simulink model "ThreePhaseInductionMachine"  (R2022b)
settings: Solver=VariableStepAuto  StartTime=0.0  StopTime=5  MaxStep=25e-6  EnableMultiTasking=on
libraries: spsACVoltageSourceLib x3, spsControlledCurrentSourceLib x3, spsVoltageMeasurementLib x3, spsSeriesRLCBranchLib x3, spsdq0toabcLib x2, spsabctodq0Lib x1, spspowerguiLib x1
settings Model: Creator=James Green  LastModifiedBy=Sarthak M Desai
settings SolverCC: AlgebraicLoopSolver=TrustRegion
settings DataIOCC: ReturnWorkspaceOutputs=off
settings OptimizationCC: LifeSpan=inf
settings DebuggingCC: UnconnectedInputMsg=warning  UnconnectedOutputMsg=warning  UnconnectedLineMsg=warning  SFUnexpectedBacktrackingDiag=warning  SFNoUnconditionalDefaultTransitionDiag=warning  SFMachineParentedDataDiag=warning  ArithmeticOperatorsInVariantConditions=warning
settings ModelReferenceCC: EnableRefExpFcnMdlSchedulingChecks=on
settings SFSimCC: SimUseLocalCustomCode=off  CustomCodeUndefinedFunction=UseInterfaceOnly
settings RTWCC: RTWUseLocalCustomCode=off
settings CodeAppCC: StateflowObjectComments=on
settings GRTTargetCC: TargetLangStandard=C89/C90 (ANSI)
settings ConfigComp: CovMetricSettings=dw  CovSaveCumulativeToWorkspaceVar=on  CovSaveSingleToWorkspaceVar=on  CovExternalEMLEnable=off
settings SimscapeCC: SimscapeNormalizeSystem=off

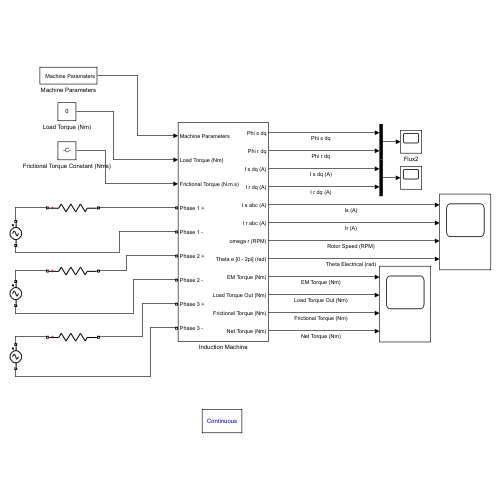
[thumbnail: Simulink's stored preview of the top-level diagram]
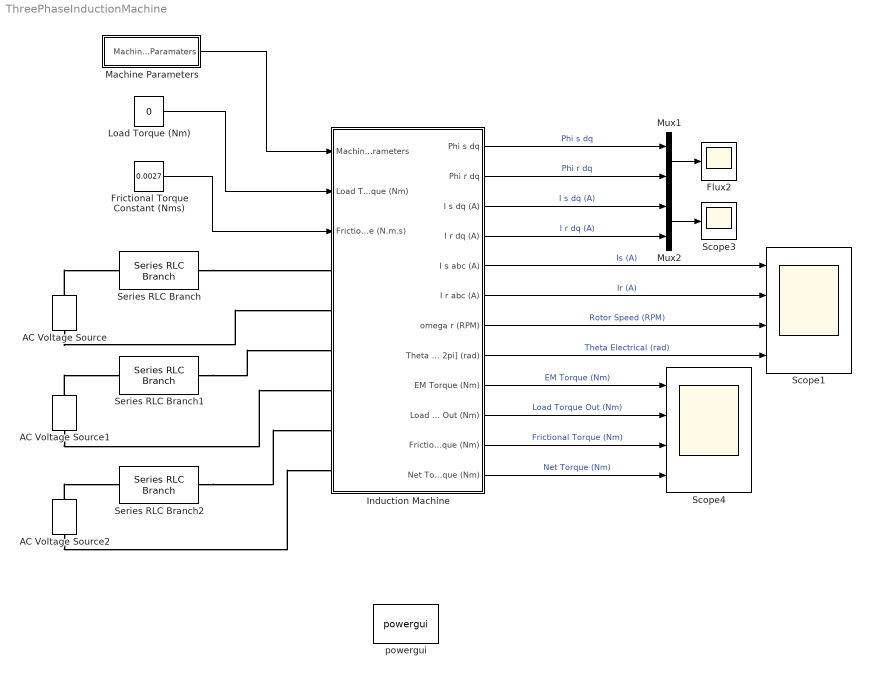
== system ThreePhaseInductionMachine ==
  AC Voltage Source : spsACVoltageSourceLib/AC Voltage Source  Amplitude=340  Phase=0  Frequency=50  SampleTime=0  Measurements=None  BusType=swing  Pref=10e3  Qref=0  Qmin=-inf  Qmax=+inf
  AC Voltage Source1 : spsACVoltageSourceLib/AC Voltage Source  Amplitude=340  Phase=-120  Frequency=50  SampleTime=0  Measurements=None  BusType=swing  Pref=10e3  Qref=0  Qmin=-inf  Qmax=+inf
  AC Voltage Source2 : spsACVoltageSourceLib/AC Voltage Source  Amplitude=340  Phase=120  Frequency=50  SampleTime=0  Measurements=None  BusType=swing  Pref=10e3  Qref=0  Qmin=-inf  Qmax=+inf
  Flux2 : Scope
  Frictional Torque Constant (Nms) : Constant  Value=0.0027
  Induction Machine : Subsystem
  Load Torque (Nm) : Constant  Value=0
  Machine Parameters : Subsystem
  Mux1 : Mux  Inputs=2
  Mux2 : Mux  Inputs=2
  Scope1 : Scope  NumInputPorts=4
  Scope3 : Scope
  Scope4 : Scope  NumInputPorts=4
  Series RLC Branch : spsSeriesRLCBranchLib/Series RLC Branch  LConnTagsString=__new0  RConnTagsString=__new0  BranchType=R  Resistance=0.1  Inductance=1e-3  SetiL0=off  InitialCurrent=0  Capacitance=1e-6  Setx0=off  InitialVoltage=0  Measurements=None
  Series RLC Branch1 : spsSeriesRLCBranchLib/Series RLC Branch  LConnTagsString=__new0  RConnTagsString=__new0  BranchType=R  Resistance=0.1  Inductance=1e-3  SetiL0=off  InitialCurrent=0  Capacitance=1e-6  Setx0=off  InitialVoltage=0  Measurements=None
  Series RLC Branch2 : spsSeriesRLCBranchLib/Series RLC Branch  LConnTagsString=__new0  RConnTagsString=__new0  BranchType=R  Resistance=0.1  Inductance=1e-3  SetiL0=off  InitialCurrent=0  Capacitance=1e-6  Setx0=off  InitialVoltage=0  Measurements=None
  powergui : spspowerguiLib/powergui  Priority=1  SimulationMode=Continuous  SampleTime=50e-6  frequency=60  Iterations=50  frequencyindice=50  Pbase=100e6  ErrMax=1e-4  UnitsV=kV  UnitsW=MW  buscounter=0  FunctionMessages=off  echomessages=off  EnableUseOfTLC=off  CurrentSourceSwitches=off  DisableSnubberDevices=off  DisableRonSwitches=off  DisableVfSwitches=off  DisplayEquations=off  AutomaticDiscreteSolvers=off  SolverType=Tustin/Backward Euler (TBE)  Interpol=off  ExternalGateDelay=off  methode=off  Ts=10  x0status=blocks  SPID=off  SwTol=0  HookPort=off  NonlinearTolerance=1e-4  nMaxIteration=100  ContinueOnMaxIteration=off  RestoreLinks=warning  ResistiveCurrentMeasurement=off  Frange=[0:2:500]  Ylog=off  Xlog=on  ShowGrid=off  save=off  variable=ZData  structure=0  ZoomFFT=off  StartTime=0.0  cycles=1  DisplayStyle=1  fundamental=60  FreqAxis=off  MaxFrequency=1000  frequencyindicesteady=1  RmsSteady=1  display=off
  wires:
  Mux1/1 -> Flux2/1
  Mux2/1 -> Scope3/1
  Induction Machine/1(Phi s dq) -> Mux1/1  "Phi s dq"
  Induction Machine/2(Phi r dq) -> Mux1/2  "Phi r dq"
  Induction Machine/3(I s dq (A)) -> Mux2/1  "I s dq (A)"
  Induction Machine/4(I r dq (A)) -> Mux2/2  "I r dq (A)"
  Induction Machine/5(I s abc (A)) -> Scope1/1  "Is (A)"
  Induction Machine/6(I r abc (A)) -> Scope1/2  "Ir (A)"
  Induction Machine/7(omega r (RPM)) -> Scope1/3  "Rotor Speed (RPM)"
  Induction Machine/8(Theta e [0 - 2pi] (rad)) -> Scope1/4  "Theta Electrical (rad)"
  Induction Machine/9(EM Torque (Nm)) -> Scope4/1  "EM Torque (Nm)"
  Induction Machine/10(Load Torque Out (Nm)) -> Scope4/2  "Load Torque Out (Nm)"
  Induction Machine/11(Frictional Torque (Nm)) -> Scope4/3  "Frictional Torque (Nm)"
  Induction Machine/12(Net Torque (Nm)) -> Scope4/4  "Net Torque (Nm)"
  Machine Parameters/1(Machine Paramaters) -> Induction Machine/1(Machine Parameters)
  Frictional Torque Constant (Nms)/1 -> Induction Machine/3(Frictional Torque (N.m.s))
  Load Torque (Nm)/1 -> Induction Machine/2(Load Torque (Nm))
  connections:
  AC Voltage Source/RConn1 -- Series RLC Branch/LConn1
  AC Voltage Source1/RConn1 -- Series RLC Branch1/LConn1
  AC Voltage Source2/RConn1 -- Series RLC Branch2/LConn1
  Series RLC Branch/RConn1 -- Induction Machine/LConn1
  AC Voltage Source/LConn1 -- Induction Machine/LConn2
  Series RLC Branch1/RConn1 -- Induction Machine/LConn3
  Series RLC Branch2/RConn1 -- Induction Machine/LConn5
  AC Voltage Source1/LConn1 -- Induction Machine/LConn4
  AC Voltage Source2/LConn1 -- Induction Machine/LConn6

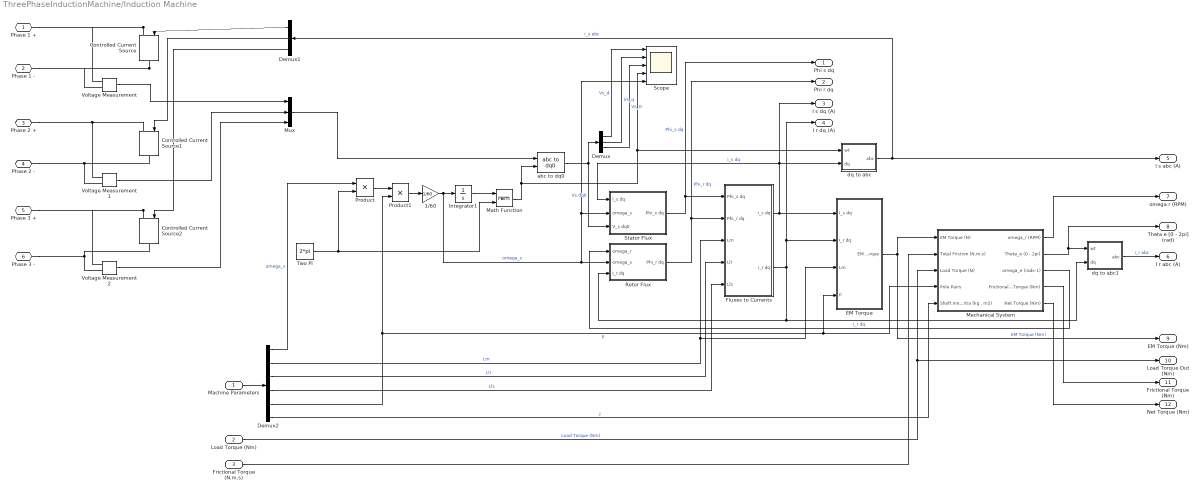
== system ThreePhaseInductionMachine/Induction Machine ==
  Machine Parameters : Inport
  Load Torque (Nm) : Inport  Port=2
  Frictional Torque (N.m.s) : Inport  Port=3
  1/60 : Gain  Gain=1/60
  Controlled Current Source : spsControlledCurrentSourceLib/Controlled Current Source  Initialize=on  Source_Type=AC  Amplitude=0  Phase=0  Frequency=0  Measurements=None
  Controlled Current Source1 : spsControlledCurrentSourceLib/Controlled Current Source  Initialize=on  Source_Type=AC  Amplitude=0  Phase=0  Frequency=0  Measurements=None
  Controlled Current Source2 : spsControlledCurrentSourceLib/Controlled Current Source  Initialize=on  Source_Type=AC  Amplitude=0  Phase=0  Frequency=0  Measurements=None
  Demux : Demux  Outputs=3
  Demux1 : Demux  Outputs=3
  Demux2 : Demux  Outputs=6
  EM Torque : Subsystem
  Fluxes to Currents : Subsystem
  Integrator1 : Integrator
  Math Function : Math  Operator=rem  SignedPower=on
  Mechanical System : Subsystem
  Mux : Mux  Inputs=3
  Product : Product
  Product1 : Product
  Rotor Flux : Subsystem
  Scope : Scope  NumInputPorts=5
  Stator Flux : Subsystem
  Two Pi : Constant  Value=2*pi
  Voltage Measurement : spsVoltageMeasurementLib/Voltage Measurement  PhasorSimulation=off  OutputType=Complex  PSBequivalent=0
  Voltage Measurement1 : spsVoltageMeasurementLib/Voltage Measurement  PhasorSimulation=off  OutputType=Complex  PSBequivalent=0
  Voltage Measurement2 : spsVoltageMeasurementLib/Voltage Measurement  PhasorSimulation=off  OutputType=Complex  PSBequivalent=0
  abc to dq0 : spsabctodq0Lib/abc to dq0  Alignment=90 degrees behind phase A axis
  dq to abc : Subsystem
  dq to abc1 : Subsystem
  Phase 1 + : PMIOPort  Side=Left
  Phase 1 - : PMIOPort  Port=2  Side=Left
  Phase 2 + : PMIOPort  Port=3  Side=Left
  Phase 2 - : PMIOPort  Port=4  Side=Left
  Phase 3 + : PMIOPort  Port=5  Side=Left
  Phase 3 - : PMIOPort  Port=6  Side=Left
  Phi s dq : Outport
  Phi r dq : Outport  Port=2
  I s dq (A) : Outport  Port=3
  I r dq (A) : Outport  Port=4
  I s abc (A) : Outport  Port=5
  I r abc (A) : Outport  Port=6
  omega r (RPM) : Outport  Port=7
  Theta e [0 - 2pi] (rad) : Outport  Port=8
  EM Torque (Nm) : Outport  Port=9
  Load Torque Out (Nm) : Outport  Port=10
  Frictional Torque (Nm) : Outport  Port=11
  Net Torque (Nm) : Outport  Port=12
  wires:
  dq to abc1/1(abc) -> I r abc (A)/1  "i_r abc"
  abc to dq0/1 -> Stator Flux/3(V_s dq0), Demux/1  "Vs dq0"
  Rotor Flux/1(Phi_r dq) -> Fluxes to Currents/2(Phi_r dq), Phi r dq/1  "Phi_r dq"
  Fluxes to Currents/1(i_s dq) -> EM Torque/1(I_s dq), Stator Flux/1(I_s dq), I s dq (A)/1, dq to abc/2(dq)  "i_s dq"
  Fluxes to Currents/2(i_r dq) -> EM Torque/2(I_r dq), I r dq (A)/1, Rotor Flux/3(I_r dq), dq to abc1/2(dq)  "i_r dq"
  Demux/3 -> Scope/3  "Vs_0"
  Demux/1 -> Scope/1  "Vs_d"
  Two Pi/1 -> Math Function/2, Product/2
  dq to abc/1(abc) -> Demux1/1, I s abc (A)/1  "i_s abc"
  Stator Flux/1(Phi_s dq) -> Fluxes to Currents/1(Phi_s dq), Phi s dq/1  "Phi_s dq"
  Load Torque (Nm)/1 -> Load Torque Out (Nm)/1, Mechanical System/3(Load Torque (N))  "Load Torque (Nm)"
  EM Torque/1(EM Torque) -> Mechanical System/1(EM Torque (N)), EM Torque (Nm)/1  "EM Torque (Nm)"
  Product1/1 -> 1/60/1
  Demux2/5 -> Product1/2, Mechanical System/4(Pole Pairs), EM Torque/4(P)  "P"
  Integrator1/1 -> Math Function/1
  Demux/2 -> Scope/2  "Vs_q"
  Voltage Measurement1/1 -> Mux/2
  Mechanical System/1(omega_r (RPM)) -> omega r (RPM)/1
  Mechanical System/2(Theta_e (0 - 2pi)) -> Theta e [0 - 2pi] (rad)/1, dq to abc1/1(wt)
  Product/1 -> Product1/1
  Mechanical System/3(omega_e (rads-1)) -> Rotor Flux/1(omega_r)
  Mechanical System/4(Frictional Torque (Nm)) -> Frictional Torque (Nm)/1
  Mechanical System/5(Net Torque (Nm)) -> Net Torque (Nm)/1
  Frictional Torque (N.m.s)/1 -> Mechanical System/2(Total Friction (N.m.s))
  1/60/1 -> Integrator1/1, Scope/5, Stator Flux/2(omega_s), Rotor Flux/2(omega_s)  "omega_s"
  Math Function/1 -> abc to dq0/2, Scope/4, dq to abc/1(wt)
  Demux1/2 -> Controlled Current Source1/1
  Demux1/1 -> Controlled Current Source/1
  Demux1/3 -> Controlled Current Source2/1
  Mux/1 -> abc to dq0/1
  Demux2/1 -> Product/1  "omega_s"
  Demux2/2 -> EM Torque/3(Lm), Fluxes to Currents/3(Lm)  "Lm"
  Demux2/3 -> Fluxes to Currents/4(Llr)  "Llr"
  Demux2/4 -> Fluxes to Currents/5(Lls)  "Lls"
  Machine Parameters/1 -> Demux2/1
  Demux2/6 -> Mechanical System/5(Shaft Innertia (kg . m2))  "J"
  Voltage Measurement/1 -> Mux/1
  Voltage Measurement2/1 -> Mux/3
  connections:
  Controlled Current Source/RConn1 -- Phase 1 -/RConn1 -- Voltage Measurement/LConn2
  Voltage Measurement1/LConn2 -- Phase 2 -/RConn1 -- Controlled Current Source1/RConn1
  Voltage Measurement1/LConn1 -- Phase 2 +/RConn1 -- Controlled Current Source1/LConn1
  Controlled Current Source2/LConn1 -- Phase 3 +/RConn1 -- Voltage Measurement2/LConn1
  Voltage Measurement2/LConn2 -- Phase 3 -/RConn1 -- Controlled Current Source2/RConn1
  Controlled Current Source/LConn1 -- Phase 1 +/RConn1 -- Voltage Measurement/LConn1

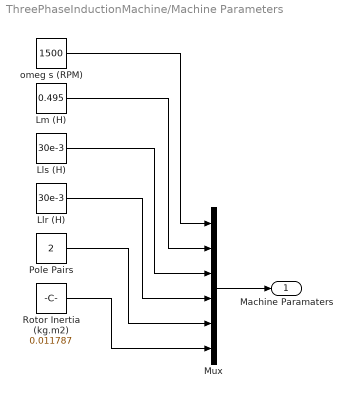
== system ThreePhaseInductionMachine/Machine Parameters ==
  Llr (H) : Constant  Value=30e-3
  Lls (H) : Constant  Value=30e-3
  Lm (H) : Constant  Value=0.495
  Mux : Mux  Inputs=6
  Pole Pairs : Constant  Value=2
  Rotor Inertia (kg.m2) : Constant  Value=0.011787
  "omeg s (RPM) " : Constant  Value=1500
  Machine Paramaters : Outport
  wires:
  Lls (H)/1 -> Mux/3
  Rotor Inertia (kg.m2)/1 -> Mux/6
  Llr (H)/1 -> Mux/4
  Pole Pairs/1 -> Mux/5
  Lm (H)/1 -> Mux/2
  Mux/1 -> Machine Paramaters/1
  "omeg s (RPM) "/1 -> Mux/1

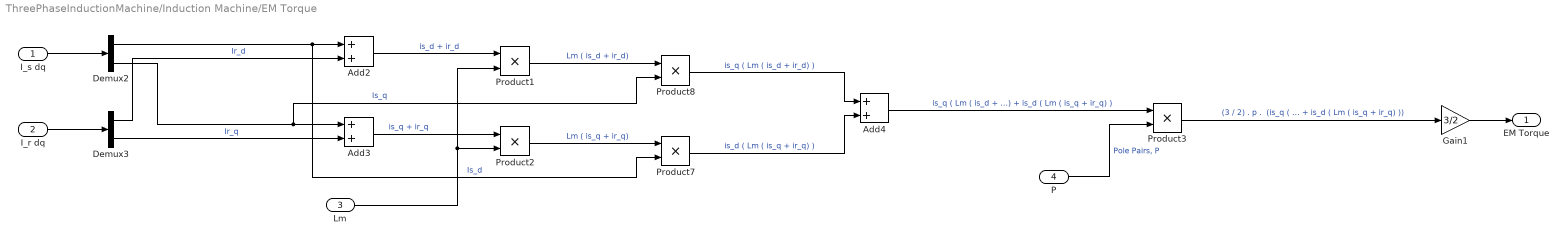
== system ThreePhaseInductionMachine/Induction Machine/EM Torque ==
  I_s dq : Inport
  I_r dq : Inport  Port=2
  Lm : Inport  Port=3
  P : Inport  Port=4
  Add2 : Sum
  Add3 : Sum
  Add4 : Sum
  Demux2 : Demux  Outputs=2
  Demux3 : Demux  Outputs=2
  Gain1 : Gain  Gain=3/2
  Product{1..3,7..8} (5 alike) : Product
  EM Torque : Outport
  wires:
  Lm/1 -> Product1/2, Product2/2
  I_r dq/1 -> Demux3/1
  Product3/1 -> Gain1/1  "(3 / 2) . p .  (is_q ( Lm ( is_d + ir_d) ) + is_d ( Lm ( is_q + ir_q) ))"
  Demux2/2 -> Product8/2, Add3/1  "Is_q"
  I_s dq/1 -> Demux2/1
  Demux3/1 -> Add2/2  "Ir_d"
  Demux3/2 -> Add3/2  "Ir_q"
  Demux2/1 -> Product7/2, Add2/1  "Is_d"
  Gain1/1 -> EM Torque/1
  Add2/1 -> Product1/1  "is_d + ir_d"
  Add3/1 -> Product2/1  "is_q + ir_q"
  Product2/1 -> Product7/1  "Lm ( is_q + ir_q)"
  Product7/1 -> Add4/2  "is_d ( Lm ( is_q + ir_q) )"
  Product1/1 -> Product8/1  "Lm ( is_d + ir_d)"
  Product8/1 -> Add4/1  "is_q ( Lm ( is_d + ir_d) )"
  Add4/1 -> Product3/1  "is_q ( Lm ( is_d + ir_d) ) + is_d ( Lm ( is_q + ir_q) )"
  P/1 -> Product3/2  "Pole Pairs, P"

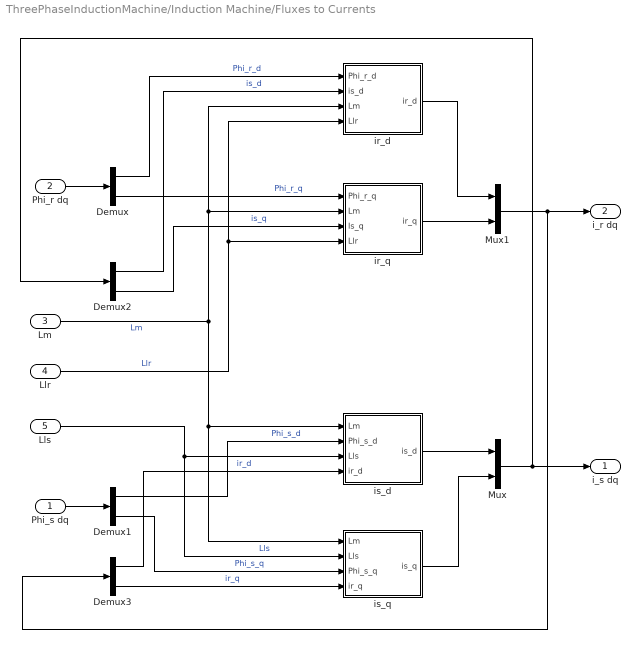
== system ThreePhaseInductionMachine/Induction Machine/Fluxes to Currents ==
  Phi_s dq : Inport
  Phi_r dq : Inport  Port=2
  Lm : Inport  Port=3
  Llr : Inport  Port=4
  Lls : Inport  Port=5
  Demux{,1..3} (4 alike) : Demux  Outputs=2
  Mux : Mux  Inputs=2
  Mux1 : Mux  Inputs=2
  ir_d : Subsystem
  ir_q : Subsystem
  is_d : Subsystem
  is_q : Subsystem
  i_s dq : Outport
  i_r dq : Outport  Port=2
  wires:
  Lls/1 -> is_q/2(Lls), is_d/3(Lls)  "Lls"
  Llr/1 -> ir_d/4(Llr), ir_q/4(Llr)  "Llr"
  Lm/1 -> is_q/1(Lm), is_d/1(Lm), ir_d/3(Lm), ir_q/2(Lm)  "Lm"
  Phi_r dq/1 -> Demux/1
  Phi_s dq/1 -> Demux1/1
  Mux/1 -> i_s dq/1, Demux2/1
  Mux1/1 -> i_r dq/1, Demux3/1
  Demux/2 -> ir_q/1(Phi_r_q)  "Phi_r_q"
  Demux2/2 -> ir_q/3(Is_q)  "is_q"
  ir_q/1(ir_q) -> Mux1/2
  Demux/1 -> ir_d/1(Phi_r_d)  "Phi_r_d"
  Demux2/1 -> ir_d/2(is_d)  "is_d"
  ir_d/1(ir_d) -> Mux1/1
  Demux1/1 -> is_d/2(Phi_s_d)  "Phi_s_d"
  Demux3/1 -> is_d/4(ir_d)  "ir_d"
  is_d/1(is_d) -> Mux/1
  Demux1/2 -> is_q/3(Phi_s_q)  "Phi_s_q"
  Demux3/2 -> is_q/4(ir_q)  "ir_q"
  is_q/1(is_q) -> Mux/2

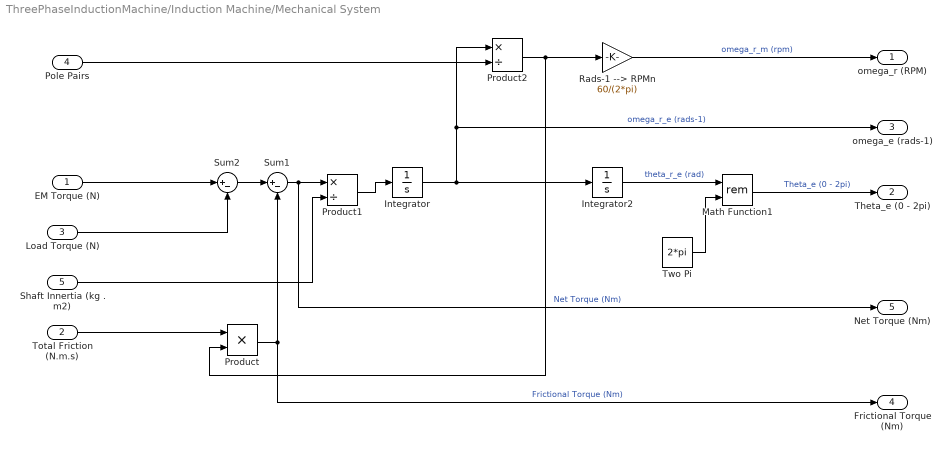
== system ThreePhaseInductionMachine/Induction Machine/Mechanical System ==
  EM Torque (N) : Inport
  Total Friction (N.m.s) : Inport  Port=2
  Load Torque (N) : Inport  Port=3
  Pole Pairs : Inport  Port=4
  Shaft Innertia (kg . m2) : Inport  Port=5
  Integrator : Integrator
  Integrator2 : Integrator
  Math Function1 : Math  Operator=rem  SignedPower=on
  Product : Product
  Product1 : Product  Inputs=*/
  Product2 : Product  Inputs=*/
  Rads-1 --> RPMn : Gain  Gain=60/(2*pi)
  Sum1 : Sum  Inputs=|+-
  Sum2 : Sum  Inputs=|+-
  Two Pi : Constant  Value=2*pi
  omega_r (RPM) : Outport
  Theta_e (0 - 2pi) : Outport  Port=2
  omega_e (rads-1) : Outport  Port=3
  Frictional Torque (Nm) : Outport  Port=4
  Net Torque (Nm) : Outport  Port=5
  wires:
  Product2/1 -> Product/2, Rads-1 --> RPMn/1
  Product1/1 -> Integrator/1
  Integrator/1 -> Product2/1, omega_e (rads-1)/1, Integrator2/1  "omega_r_e (rads-1)"
  Two Pi/1 -> Math Function1/2
  Integrator2/1 -> Math Function1/1  "theta_r_e (rad)"
  Math Function1/1 -> Theta_e (0 - 2pi)/1  "Theta_e (0 - 2pi)"
  EM Torque (N)/1 -> Sum2/1
  Load Torque (N)/1 -> Sum2/2
  Rads-1 --> RPMn/1 -> omega_r (RPM)/1  "omega_r_m (rpm)"
  Sum2/1 -> Sum1/1
  Product/1 -> Sum1/2, Frictional Torque (Nm)/1  "Frictional Torque (Nm)"
  Total Friction (N.m.s)/1 -> Product/1
  Sum1/1 -> Product1/1, Net Torque (Nm)/1  "Net Torque (Nm)"
  Pole Pairs/1 -> Product2/2
  Shaft Innertia (kg . m2)/1 -> Product1/2

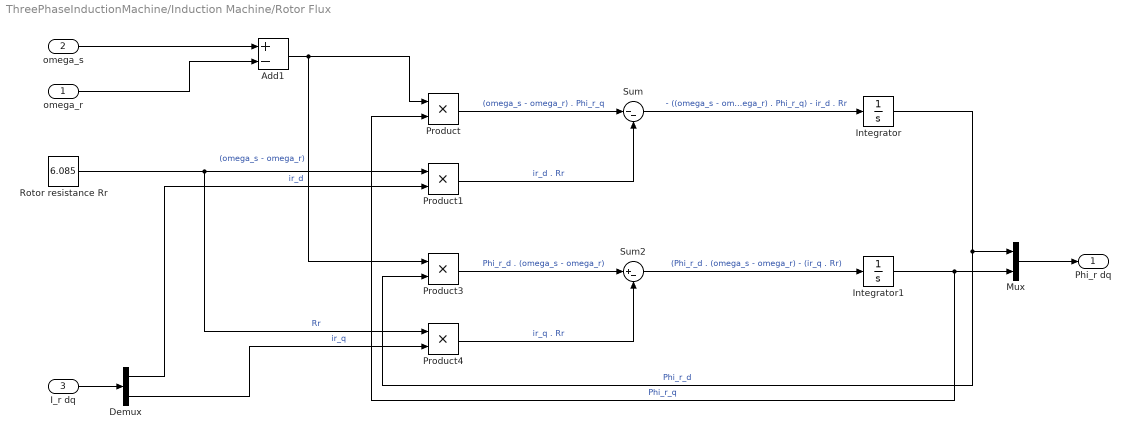
== system ThreePhaseInductionMachine/Induction Machine/Rotor Flux ==
  omega_r : Inport
  omega_s : Inport  Port=2
  I_r dq : Inport  Port=3
  Add1 : Sum  Inputs=+-
  Demux : Demux  Outputs=2
  Integrator : Integrator
  Integrator1 : Integrator
  Mux : Mux  Inputs=2
  Product{,1,3..4} (4 alike) : Product
  Rotor resistance Rr : Constant  Value=6.085
  Sum : Sum  Inputs=|--
  Sum2 : Sum  Inputs=|+-
  Phi_r dq : Outport
  wires:
  Product3/1 -> Sum2/1  "Phi_r_d . (omega_s - omega_r)"
  omega_r/1 -> Add1/2
  Rotor resistance Rr/1 -> Product1/1, Product4/1  "Rr"
  Integrator1/1 -> Product/2, Mux/2  "Phi_r_q"
  Sum2/1 -> Integrator1/1  "(Phi_r_d . (omega_s - omega_r) - (ir_q . Rr)"
  Demux/2 -> Product4/2  "ir_q"
  Product1/1 -> Sum/2  "ir_d . Rr"
  Product4/1 -> Sum2/2  "ir_q . Rr"
  omega_s/1 -> Add1/1
  Product/1 -> Sum/1  "(omega_s - omega_r) . Phi_r_q"
  Add1/1 -> Product/1, Product3/1  "(omega_s - omega_r)"
  Integrator/1 -> Product3/2, Mux/1  "Phi_r_d"
  Sum/1 -> Integrator/1  "- ((omega_s - omega_r) . Phi_r_q) - ir_d . Rr"
  I_r dq/1 -> Demux/1
  Demux/1 -> Product1/2  "ir_d"
  Mux/1 -> Phi_r dq/1

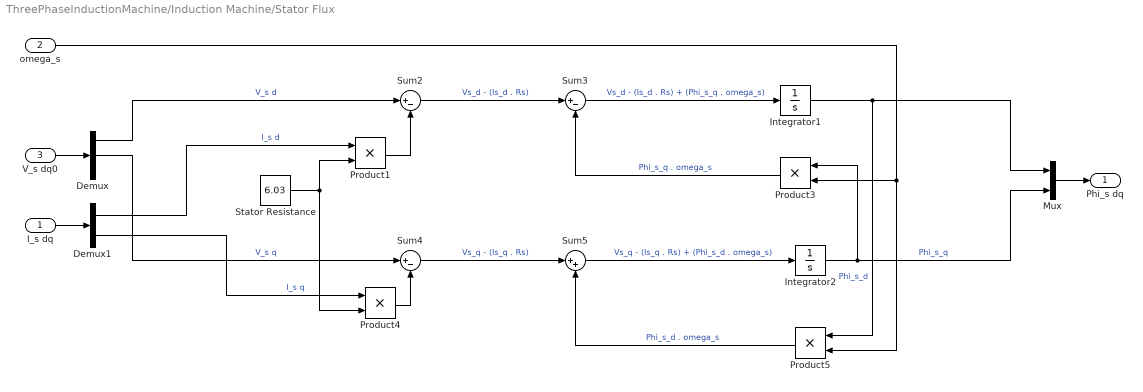
== system ThreePhaseInductionMachine/Induction Machine/Stator Flux ==
  I_s dq : Inport
  omega_s : Inport  Port=2
  V_s dq0 : Inport  Port=3
  Demux : Demux  Outputs=3
  Demux1 : Demux  Outputs=2
  Integrator1 : Integrator
  Integrator2 : Integrator
  Mux : Mux  Inputs=2
  Product{1,3..5} (4 alike) : Product
  Stator Resistance : Constant  Value=6.03
  Sum2 : Sum  Inputs=|+-
  Sum3 : Sum  Inputs=|+-
  Sum4 : Sum  Inputs=|+-
  Sum5 : Sum  Inputs=|++
  Phi_s dq : Outport
  wires:
  Sum2/1 -> Sum3/1  "Vs_d - (Is_d . Rs)"
  Demux1/1 -> Product1/1  "I_s d"
  Product3/1 -> Sum3/2  "Phi_s_q . omega_s"
  Sum3/1 -> Integrator1/1  "Vs_d - (Is_d . Rs) + (Phi_s_q . omega_s)"
  Demux/1 -> Sum2/1  "V_s d"
  Demux/2 -> Sum4/1  "V_s q"
  Product4/1 -> Sum4/2
  Integrator1/1 -> Product5/1, Mux/1  "Phi_s_d"
  Demux1/2 -> Product4/1  "I_s q"
  Sum4/1 -> Sum5/1  "Vs_q - (Is_q . Rs)"
  omega_s/1 -> Product5/2, Product3/2
  Product1/1 -> Sum2/2
  Integrator2/1 -> Product3/1, Mux/2  "Phi_s_q"
  Product5/1 -> Sum5/2  "Phi_s_d . omega_s"
  Stator Resistance/1 -> Product4/2, Product1/2
  Sum5/1 -> Integrator2/1  "Vs_q - (Is_q . Rs) + (Phi_s_d . omega_s)"
  Mux/1 -> Phi_s dq/1
  I_s dq/1 -> Demux1/1
  V_s dq0/1 -> Demux/1

== system ThreePhaseInductionMachine/Induction Machine/dq to abc ==
  wt : Inport
  dq : Inport  Port=2
  Constant1 : Constant  Value=0
  Demux1 : Demux  Outputs=2
  Mux1 : Mux  Inputs=3
  dq0 to abc : spsdq0toabcLib/dq0 to abc  Alignment=90 degrees behind phase A axis
  abc : Outport
  wires:
  Mux1/1 -> dq0 to abc/1
  Demux1/2 -> Mux1/2
  wt/1 -> dq0 to abc/2
  dq/1 -> Demux1/1
  dq0 to abc/1 -> abc/1
  Constant1/1 -> Mux1/3
  Demux1/1 -> Mux1/1

== system ThreePhaseInductionMachine/Induction Machine/dq to abc1 ==
  wt : Inport
  dq : Inport  Port=2
  Constant1 : Constant  Value=0
  Demux1 : Demux  Outputs=2
  Mux1 : Mux  Inputs=3
  dq0 to abc : spsdq0toabcLib/dq0 to abc  Alignment=90 degrees behind phase A axis
  abc : Outport
  wires:
  Demux1/1 -> Mux1/1
  Constant1/1 -> Mux1/3
  dq0 to abc/1 -> abc/1
  dq/1 -> Demux1/1
  wt/1 -> dq0 to abc/2
  Demux1/2 -> Mux1/2
  Mux1/1 -> dq0 to abc/1

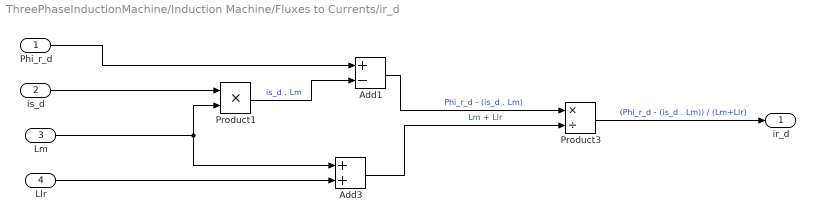
== system ThreePhaseInductionMachine/Induction Machine/Fluxes to Currents/ir_d ==
  Phi_r_d : Inport
  is_d : Inport  Port=2
  Lm : Inport  Port=3
  Llr : Inport  Port=4
  Add1 : Sum  Inputs=+-
  Add3 : Sum
  Product1 : Product
  Product3 : Product  Inputs=*/
  ir_d : Outport
  wires:
  is_d/1 -> Product1/1
  Add1/1 -> Product3/1  "Phi_r_d - (is_d . Lm)"
  Add3/1 -> Product3/2  "Lm + Llr"
  Product1/1 -> Add1/2  "is_d . Lm"
  Phi_r_d/1 -> Add1/1
  Lm/1 -> Add3/1, Product1/2
  Llr/1 -> Add3/2
  Product3/1 -> ir_d/1  "(Phi_r_d - (is_d . Lm)) / (Lm+Llr)"

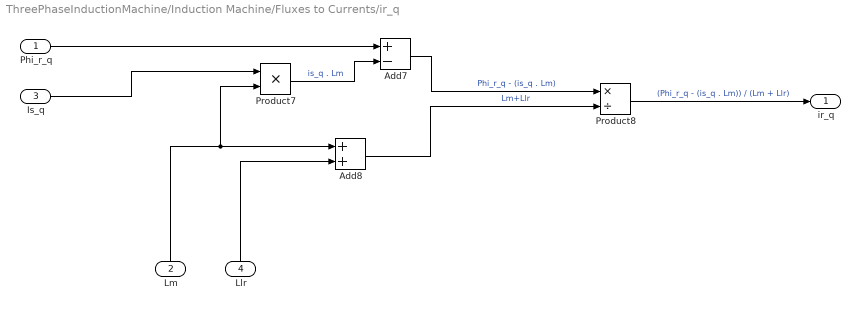
== system ThreePhaseInductionMachine/Induction Machine/Fluxes to Currents/ir_q ==
  Phi_r_q : Inport
  Lm : Inport  Port=2
  Is_q : Inport  Port=3
  Llr : Inport  Port=4
  Add7 : Sum  Inputs=+-
  Add8 : Sum
  Product7 : Product
  Product8 : Product  Inputs=*/
  ir_q : Outport
  wires:
  Lm/1 -> Product7/2, Add8/1
  Llr/1 -> Add8/2
  Product8/1 -> ir_q/1  "(Phi_r_q - (is_q . Lm)) / (Lm + Llr)"
  Product7/1 -> Add7/2  "is_q . Lm"
  Phi_r_q/1 -> Add7/1
  Add7/1 -> Product8/1  "Phi_r_q - (is_q . Lm)"
  Add8/1 -> Product8/2  "Lm+Llr"
  Is_q/1 -> Product7/1

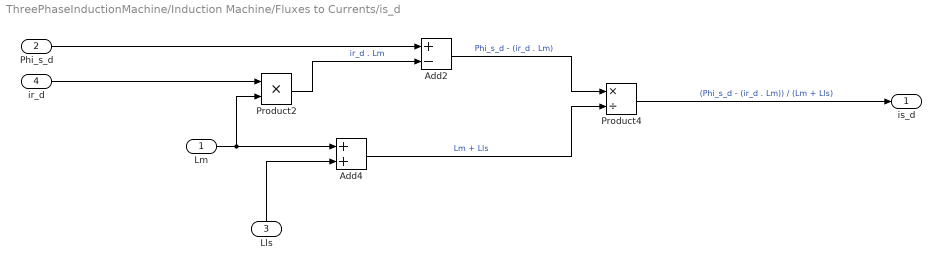
== system ThreePhaseInductionMachine/Induction Machine/Fluxes to Currents/is_d ==
  Lm : Inport
  Phi_s_d : Inport  Port=2
  Lls : Inport  Port=3
  ir_d : Inport  Port=4
  Add2 : Sum  Inputs=+-
  Add4 : Sum
  Product2 : Product
  Product4 : Product  Inputs=*/
  is_d : Outport
  wires:
  Product4/1 -> is_d/1  "(Phi_s_d - (ir_d . Lm)) / (Lm + Lls)"
  Lm/1 -> Product2/2, Add4/1
  Lls/1 -> Add4/2
  Product2/1 -> Add2/2  "ir_d . Lm"
  Phi_s_d/1 -> Add2/1
  Add4/1 -> Product4/2  "Lm + Lls"
  ir_d/1 -> Product2/1
  Add2/1 -> Product4/1  "Phi_s_d - (ir_d . Lm)"

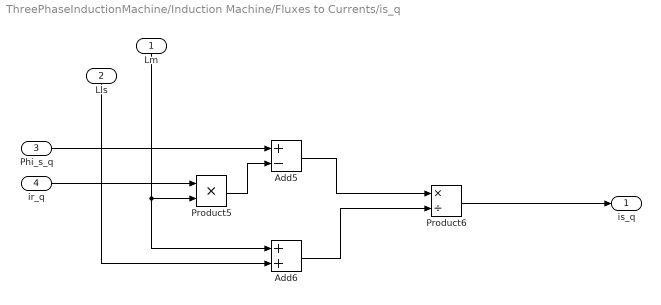
== system ThreePhaseInductionMachine/Induction Machine/Fluxes to Currents/is_q ==
  Lm : Inport
  Lls : Inport  Port=2
  Phi_s_q : Inport  Port=3
  ir_q : Inport  Port=4
  Add5 : Sum  Inputs=+-
  Add6 : Sum
  Product5 : Product
  Product6 : Product  Inputs=*/
  is_q : Outport
  wires:
  Lls/1 -> Add6/2
  Lm/1 -> Product5/2, Add6/1
  ir_q/1 -> Product5/1
  Add6/1 -> Product6/2
  Add5/1 -> Product6/1
  Phi_s_q/1 -> Add5/1
  Product6/1 -> is_q/1
  Product5/1 -> Add5/2
